simulink model "corde"  (R2019b)
settings: Solver=VariableStepAuto  StartTime=0.0  StopTime=10.0  RelTol=1e-3
libraries: simulink x1
settings Model: Creator=thomaslabbe  LastModifiedBy=thomaslabbe

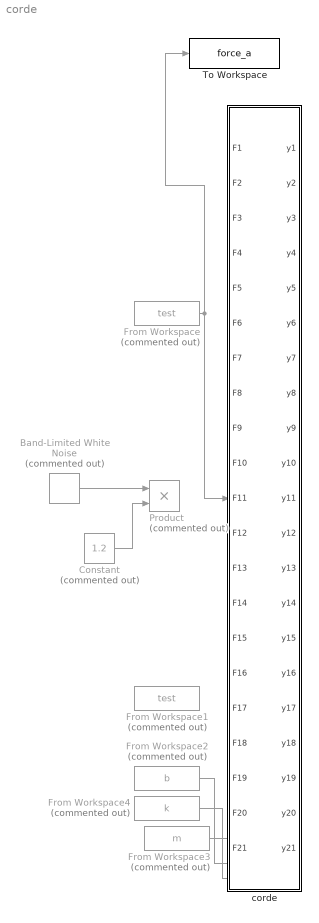
== system corde ==
  Band-Limited White Noise : simulink/Sources/Band-Limited White Noise  Commented=on  Cov=[0.1]  Ts=0.1  seed=[23341]
  Constant : Constant  Commented=on  Value=1.2
  From Workspace : FromWorkspace  Commented=on  VariableName=test  SampleTime=0
  From Workspace1 : FromWorkspace  Commented=on  VariableName=test  SampleTime=0
  From Workspace2 : FromWorkspace  Commented=on  VariableName=b  SampleTime=0
  From Workspace3 : FromWorkspace  Commented=on  VariableName=m  SampleTime=0
  From Workspace4 : FromWorkspace  Commented=on  VariableName=k  SampleTime=0
  Product : Product  Commented=on
  To Workspace : ToWorkspace  VariableName=force_a  SaveFormat=Timeseries  SampleTime=-1
  "corde " : Subsystem
  wires:
  From Workspace4/1 -> ?
  From Workspace3/1 -> ?
  From Workspace2/1 -> ?
  From Workspace/1 -> "corde "/11(F11), To Workspace/1
  Constant/1 -> Product/2
  Band-Limited White Noise/1 -> Product/1

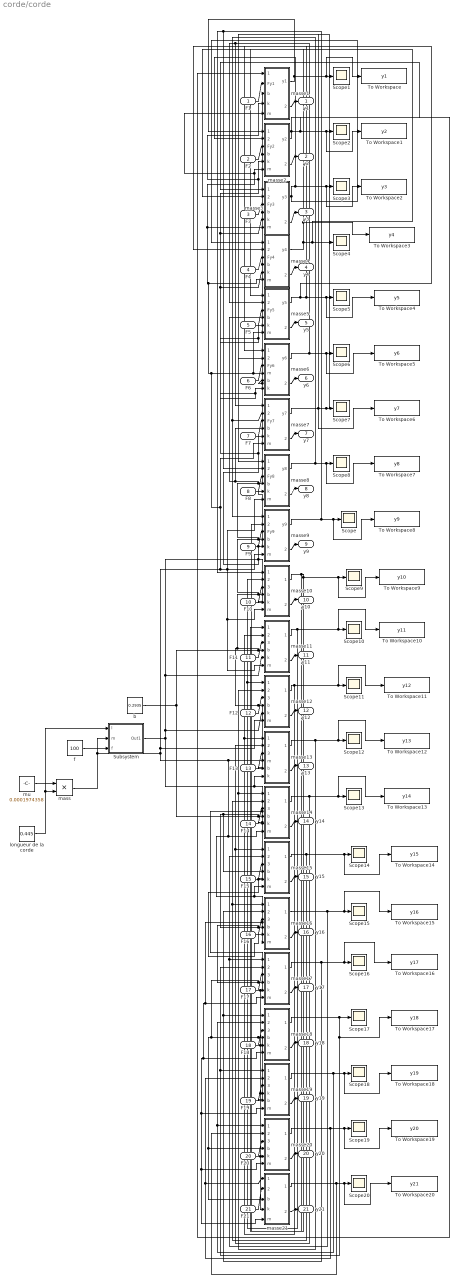
== system corde/corde  ==
  F1 : Inport
  F2 : Inport  Port=2
  F3 : Inport  Port=3
  F4 : Inport  Port=4
  F5 : Inport  Port=5
  F6 : Inport  Port=6
  F7 : Inport  Port=7
  F8 : Inport  Port=8
  F9 : Inport  Port=9
  F10 : Inport  Port=10
  F11 : Inport  Port=11
  F12 : Inport  Port=12
  F13 : Inport  Port=13
  F14 : Inport  Port=14
  F15 : Inport  Port=15
  F16 : Inport  Port=16
  F17 : Inport  Port=17
  F18 : Inport  Port=18
  F19 : Inport  Port=19
  F20 : Inport  Port=20
  F21 : Inport  Port=21
  Scope{,1..20} (21 alike) : Scope
  Subsystem : Subsystem
  To Workspace : ToWorkspace  VariableName=y1  SampleTime=-1
      settings: Save2DSignal=2-D array (concatenate along first dimension)
  To Workspace1 : ToWorkspace  VariableName=y2  SampleTime=-1
      settings: Save2DSignal=2-D array (concatenate along first dimension)
  To Workspace10 : ToWorkspace  VariableName=y11  SampleTime=-1
      settings: Save2DSignal=2-D array (concatenate along first dimension)
  To Workspace11 : ToWorkspace  VariableName=y12  SampleTime=-1
      settings: Save2DSignal=2-D array (concatenate along first dimension)
  To Workspace12 : ToWorkspace  VariableName=y13  SampleTime=-1
      settings: Save2DSignal=2-D array (concatenate along first dimension)
  To Workspace13 : ToWorkspace  VariableName=y14  SampleTime=-1
      settings: Save2DSignal=2-D array (concatenate along first dimension)
  To Workspace14 : ToWorkspace  VariableName=y15  SampleTime=-1
      settings: Save2DSignal=2-D array (concatenate along first dimension)
  To Workspace15 : ToWorkspace  VariableName=y16  SampleTime=-1
      settings: Save2DSignal=2-D array (concatenate along first dimension)
  To Workspace16 : ToWorkspace  VariableName=y17  SampleTime=-1
      settings: Save2DSignal=2-D array (concatenate along first dimension)
  To Workspace17 : ToWorkspace  VariableName=y18  SampleTime=-1
      settings: Save2DSignal=2-D array (concatenate along first dimension)
  To Workspace18 : ToWorkspace  VariableName=y19  SampleTime=-1
      settings: Save2DSignal=2-D array (concatenate along first dimension)
  To Workspace19 : ToWorkspace  VariableName=y20  SampleTime=-1
      settings: Save2DSignal=2-D array (concatenate along first dimension)
  To Workspace2 : ToWorkspace  VariableName=y3  SampleTime=-1
      settings: Save2DSignal=2-D array (concatenate along first dimension)
  To Workspace20 : ToWorkspace  VariableName=y21  SampleTime=-1
      settings: Save2DSignal=2-D array (concatenate along first dimension)
  To Workspace3 : ToWorkspace  VariableName=y4  SampleTime=-1
      settings: Save2DSignal=2-D array (concatenate along first dimension)
  To Workspace4 : ToWorkspace  VariableName=y5  SampleTime=-1
      settings: Save2DSignal=2-D array (concatenate along first dimension)
  To Workspace5 : ToWorkspace  VariableName=y6  SampleTime=-1
      settings: Save2DSignal=2-D array (concatenate along first dimension)
  To Workspace6 : ToWorkspace  VariableName=y7  SampleTime=-1
      settings: Save2DSignal=2-D array (concatenate along first dimension)
  To Workspace7 : ToWorkspace  VariableName=y8  SampleTime=-1
      settings: Save2DSignal=2-D array (concatenate along first dimension)
  To Workspace8 : ToWorkspace  VariableName=y9  SampleTime=-1
      settings: Save2DSignal=2-D array (concatenate along first dimension)
  To Workspace9 : ToWorkspace  VariableName=y10  SampleTime=-1
      settings: Save2DSignal=2-D array (concatenate along first dimension)
  b : Constant  Value=0.2935
  f : Constant  Value=100
  "longueur de la corde " : Constant  Value=0.445
  mass : Product
  masse1 : Subsystem  mask{m=0.01, k=2000, b=0.1, pos_ini=0, v_ini=0}
      mask prompts: m "Masse"; k "Force rappel d'un ressort"; b "Frottement"; pos_ini "Position initiale"; v_ini "Vitesse initiale"
  masse10 : Subsystem  mask{m=0.01, k=2000, b=0.1, pos_ini=0, v_ini=0}
      mask prompts: m "Masse"; k "Force rappel d'un ressort"; b "Frottement"; pos_ini "Position initiale"; v_ini "Vitesse initiale"
  masse11 : Subsystem  mask{m=0.01, k=2000, b=0.1, pos_ini=0, v_ini=0}
      mask prompts: m "Masse"; k "Force rappel d'un ressort"; b "Frottement"; pos_ini "Position initiale"; v_ini "Vitesse initiale"
  masse12 : Subsystem  mask{m=0.01, k=2000, b=0.1, pos_ini=0, v_ini=0}
      mask prompts: m "Masse"; k "Force rappel d'un ressort"; b "Frottement"; pos_ini "Position initiale"; v_ini "Vitesse initiale"
  masse13 : Subsystem  mask{m=0.01, k=2000, b=0.1, pos_ini=0, v_ini=0}
      mask prompts: m "Masse"; k "Force rappel d'un ressort"; b "Frottement"; pos_ini "Position initiale"; v_ini "Vitesse initiale"
  masse14 : Subsystem  mask{m=0.01, k=2000, b=0.1, pos_ini=0, v_ini=0}
      mask prompts: m "Masse"; k "Force rappel d'un ressort"; b "Frottement"; pos_ini "Position initiale"; v_ini "Vitesse initiale"
  masse15 : Subsystem  mask{m=0.01, k=2000, b=0.1, pos_ini=0, v_ini=0}
      mask prompts: m "Masse"; k "Force rappel d'un ressort"; b "Frottement"; pos_ini "Position initiale"; v_ini "Vitesse initiale"
  masse16 : Subsystem  mask{m=0.01, k=2000, b=0.1, pos_ini=0, v_ini=0}
      mask prompts: m "Masse"; k "Force rappel d'un ressort"; b "Frottement"; pos_ini "Position initiale"; v_ini "Vitesse initiale"
  masse17 : Subsystem  mask{m=0.01, k=2000, b=0.1, pos_ini=0, v_ini=0}
      mask prompts: m "Masse"; k "Force rappel d'un ressort"; b "Frottement"; pos_ini "Position initiale"; v_ini "Vitesse initiale"
  masse18 : Subsystem  mask{m=0.01, k=2000, b=0.1, pos_ini=0, v_ini=0}
      mask prompts: m "Masse"; k "Force rappel d'un ressort"; b "Frottement"; pos_ini "Position initiale"; v_ini "Vitesse initiale"
  masse19 : Subsystem  mask{m=0.01, k=2000, b=0.1, pos_ini=0, v_ini=0}
      mask prompts: m "Masse"; k "Force rappel d'un ressort"; b "Frottement"; pos_ini "Position initiale"; v_ini "Vitesse initiale"
  "masse2 " : Subsystem  mask{m=0.01, k=2000, b=0.1, pos_ini=0, v_ini=0}
      mask prompts: m "Masse"; k "Force rappel d'un ressort"; b "Frottement"; pos_ini "Position initiale"; v_ini "Vitesse initiale"
  masse20 : Subsystem  mask{m=0.01, k=2000, b=0.1, pos_ini=0, v_ini=0}
      mask prompts: m "Masse"; k "Force rappel d'un ressort"; b "Frottement"; pos_ini "Position initiale"; v_ini "Vitesse initiale"
  masse21 : Subsystem  mask{m=0.01, k=2000, b=0.1, pos_ini=0.0, v_ini=0}
      mask prompts: m "Masse"; k "Force rappel d'un ressort"; b "Frottement"; pos_ini "Position initiale"; v_ini "Vitesse initiale"
  masse3 : Subsystem  mask{m=0.01, k=2000, b=0.1, pos_ini=0, v_ini=0}
      mask prompts: m "Masse"; k "Force rappel d'un ressort"; b "Frottement"; pos_ini "Position initiale"; v_ini "Vitesse initiale"
  masse4 : Subsystem  mask{m=0.01, k=2000, b=0.1, pos_ini=0, v_ini=0}
      mask prompts: m "Masse"; k "Force rappel d'un ressort"; b "Frottement"; pos_ini "Position initiale"; v_ini "Vitesse initiale"
  masse5 : Subsystem  mask{m=0.01, k=2000, b=0.1, pos_ini=0, v_ini=0}
      mask prompts: m "Masse"; k "Force rappel d'un ressort"; b "Frottement"; pos_ini "Position initiale"; v_ini "Vitesse initiale"
  masse6 : Subsystem  mask{m=0.01, k=2000, b=0.1, pos_ini=0, v_ini=0}
      mask prompts: m "Masse"; k "Force rappel d'un ressort"; b "Frottement"; pos_ini "Position initiale"; v_ini "Vitesse initiale"
  masse7 : Subsystem  mask{m=0.01, k=2000, b=0.1, pos_ini=0, v_ini=0}
      mask prompts: m "Masse"; k "Force rappel d'un ressort"; b "Frottement"; pos_ini "Position initiale"; v_ini "Vitesse initiale"
  masse8 : Subsystem  mask{m=0.01, k=2000, b=0.1, pos_ini=0, v_ini=0}
      mask prompts: m "Masse"; k "Force rappel d'un ressort"; b "Frottement"; pos_ini "Position initiale"; v_ini "Vitesse initiale"
  masse9 : Subsystem  mask{m=0.01, k=2000, b=0.1, pos_ini=0, v_ini=0}
      mask prompts: m "Masse"; k "Force rappel d'un ressort"; b "Frottement"; pos_ini "Position initiale"; v_ini "Vitesse initiale"
  mu : Constant  Value=0.0001974358
  y1 : Outport
  y2 : Outport  Port=2
  y3 : Outport  Port=3
  y4 : Outport  Port=4
  y5 : Outport  Port=5
  y6 : Outport  Port=6
  y7 : Outport  Port=7
  y8 : Outport  Port=8
  y9 : Outport  Port=9
  y10 : Outport  Port=10
  y11 : Outport  Port=11
  y12 : Outport  Port=12
  y13 : Outport  Port=13
  y14 : Outport  Port=14
  y15 : Outport  Port=15
  y16 : Outport  Port=16
  y17 : Outport  Port=17
  y18 : Outport  Port=18
  y19 : Outport  Port=19
  y20 : Outport  Port=20
  y21 : Outport  Port=21
  wires:
  masse20/2(vy20) -> y20/1
  masse8/2(vy8) -> y8/1
  masse4/2(vy4) -> y4/1
  masse17/2(vy17) -> y17/1
  F17/1 -> masse17/3(Fy17)
  F1/1 -> masse1/2(Fy1)
  F5/1 -> masse5/3(Fy5)
  masse7/2(vy7) -> y7/1
  masse19/2(vy19) -> y19/1
  "masse2 "/2(vy2) -> y2/1
  F21/1 -> masse21/2(Fy21)
  F10/1 -> masse10/3(Fy10)
  masse15/1(y15) -> To Workspace14/1, Scope14/1, masse16/1(yp15), masse14/2(yp15)
  F11/1 -> masse11/3(Fy11)
  F6/1 -> masse6/3(Fy6)
  F15/1 -> masse15/3(Fy15)
  masse1/2(vy1) -> y1/1
  masse10/2(vy10) -> y10/1
  "masse2 "/1(y2) -> masse3/1(yp2), To Workspace1/1, Scope2/1, masse1/1(yp2)
  F2/1 -> "masse2 "/3(Fy2)
  F14/1 -> masse14/3(Fy14)
  masse17/1(y17) -> To Workspace16/1, Scope16/1, masse18/1(yp17), masse16/2(yp17)
  masse12/2(vy12) -> y12/1
  F4/1 -> masse4/3(Fy4)
  masse6/2(vy6) -> y6/1
  masse19/1(y19) -> To Workspace18/1, Scope18/1, masse20/1(yp19), masse18/2(yp19)
  masse5/1(y5) -> masse4/2(yp5), To Workspace4/1, Scope5/1, masse6/1(yp5)
  masse3/2(vy3) -> y3/1
  masse16/2(vy16) -> y16/1
  masse11/2(vy11) -> y11/1
  masse13/1(y13) -> To Workspace12/1, Scope12/1, masse14/1(yp13), masse12/2(yp13)
  masse12/1(y12) -> To Workspace11/1, Scope11/1, masse13/1(yp12), masse11/2(yp12)
  F20/1 -> masse20/3(Fy20)
  F18/1 -> masse18/3(Fy18)
  masse18/2(vy18) -> y18/1
  masse8/1(y8) -> To Workspace7/1, Scope8/1, masse9/1(yp8), masse7/2(yp8)
  masse21/2(vy21) -> y21/1
  masse9/2(vy9) -> y9/1
  masse14/1(y14) -> To Workspace13/1, Scope13/1, masse15/1(yp14), masse13/2(yp14)
  masse20/1(y20) -> To Workspace19/1, Scope19/1, masse21/1(yp20), masse19/2(yp20)
  F19/1 -> masse19/3(Fy19)
  masse16/1(y16) -> To Workspace15/1, Scope15/1, masse17/1(yp16), masse15/2(yp16)
  masse9/1(y9) -> masse8/2(yp9), masse10/1(yp9), To Workspace8/1, Scope/1
  masse5/2(vy5) -> y5/1
  masse11/1(y11) -> To Workspace10/1, Scope10/1, masse12/1(yp11), masse10/2(yp11)
  masse3/1(y3) -> To Workspace2/1, Scope3/1, "masse2 "/2(yp3), masse4/1(yp3)
  masse21/1(y21) -> To Workspace20/1, Scope20/1, masse20/2(yp21)
  F8/1 -> masse8/3(Fy8)
  masse13/2(vy13) -> y13/1
  F9/1 -> masse9/3(Fy9)
  masse10/1(y10) -> masse9/2(yp10), To Workspace9/1, Scope9/1, masse11/1(yp10)
  F16/1 -> masse16/3(Fy16)
  masse18/1(y18) -> masse19/1(yp18), masse17/2(yp18), To Workspace17/1, Scope17/1
  masse6/1(y6) -> masse7/1(yp6), masse5/2(yp6), To Workspace5/1, Scope6/1
  F7/1 -> masse7/3(Fy7)
  F13/1 -> masse13/3(Fy13)
  masse4/1(y4) -> masse5/1(yp4), To Workspace3/1, masse3/2(yp4), Scope4/1
  F12/1 -> masse12/3(Fy12)
  masse15/2(vy15) -> y15/1
  F3/1 -> masse3/3(Fy3)
  masse7/1(y7) -> masse6/2(yp7), Scope7/1, masse8/1(yp7), To Workspace6/1
  masse14/2(vy14) -> y14/1
  masse1/1(y1) -> To Workspace/1, Scope1/1, "masse2 "/1(yp1)
  b/1 -> masse15/4(b), masse19/5(b), masse18/4(b), masse20/4(b), masse21/3(b), masse17/4(b), masse16/4(b), masse14/4(b), masse6/5("b "), masse1/3(b), "masse2 "/4(b), masse3/4(b), masse4/4(b), masse7/4(b), masse5/4("b "), masse8/4(b), masse9/4(b), masse10/4(b), masse13/5(b), masse12/4(b), masse11/4(b)
  mass/1 -> Subsystem/2(m), masse7/6(m), masse6/4(m), masse5/6(m), masse4/6(m), masse3/6(m), "masse2 "/6(m), masse1/5(m), masse10/6(m), masse11/6(m), masse9/6(m), masse8/6(m), masse12/6(m), masse13/4(m), masse14/6(m), masse16/6(m), masse17/6(m), masse18/6(m), masse19/6(m), masse20/6(m), masse21/5(m), masse15/6(m)
  Subsystem/1(Out1) -> masse8/5(k), masse9/5(k), masse7/5(k), masse6/6(k), masse5/5(k), masse4/5(k), masse3/5(k), "masse2 "/5(k), masse1/4(k), masse10/5(k), masse11/5(k), masse12/5(k), masse14/5("k "), masse16/5(k), masse15/5(k), masse21/4(k), masse20/5(k), masse19/4(k), masse18/5(k), masse17/5(k), masse13/6(k)
  f/1 -> Subsystem/3(f)
  "longueur de la corde "/1 -> Subsystem/1(l), mass/2
  mu/1 -> mass/1

== system corde/corde /Subsystem ==
  l : Inport
  m : Inport  Port=2
  f : Inport  Port=3
  Divide : Product  Inputs=*/
  Divide1 : Product  Inputs=*/
  Sqrt : Sqrt  SaturateOnIntegerOverflow=on
  Tension : Polyval  Coefs=[1.138, -56.541]
  Out1 : Outport
  wires:
  Sqrt/1 -> Out1/1
  f/1 -> Tension/1
  Divide1/1 -> Sqrt/1
  Tension/1 -> Divide/1
  l/1 -> Divide/2
  Divide/1 -> Divide1/1
  m/1 -> Divide1/2

== system corde/corde /masse1 ==
  yp2 : Inport
  Fy1 : Inport  Port=2
  b : Inport  Port=3
  k : Inport  Port=4
  m : Inport  Port=5
  " " : Gain  Gain=2  SaturateOnIntegerOverflow=on  OutDataTypeStr=Inherit: Same as input  ParamDataTypeStr=Inherit: Same as input
  Divide : Product  Inputs=*/
  Position y1 : Integrator  InitialCondition=pos_ini
  Product1 : Product
  Product2 : Product
  Somme Force : Sum  Inputs=++-  SaturateOnIntegerOverflow=on  InputSameDT=on  OutDataTypeStr=Inherit: Same as first input
  Somme y : Sum  Inputs=-+  SaturateOnIntegerOverflow=on  InputSameDT=on  OutDataTypeStr=Inherit: Same as first input
  Vitesse y1 : Integrator  InitialCondition=v_ini
  y1 : Outport  VectorParamsAs1DForOutWhenUnconnected=off
  vy1 : Outport  Port=2  VectorParamsAs1DForOutWhenUnconnected=off
  wires:
  Position y1/1 -> " "/1, y1/1
  Vitesse y1/1 -> Position y1/1, Product2/2, vy1/1
  Divide/1 -> Vitesse y1/1
  Somme Force/1 -> Divide/1
  Product1/1 -> Somme Force/1
  Somme y/1 -> Product1/2
  Product2/1 -> Somme Force/3
  Fy1/1 -> Somme Force/2
  yp2/1 -> Somme y/2
  " "/1 -> Somme y/1
  b/1 -> Product2/1
  k/1 -> Product1/1
  m/1 -> Divide/2

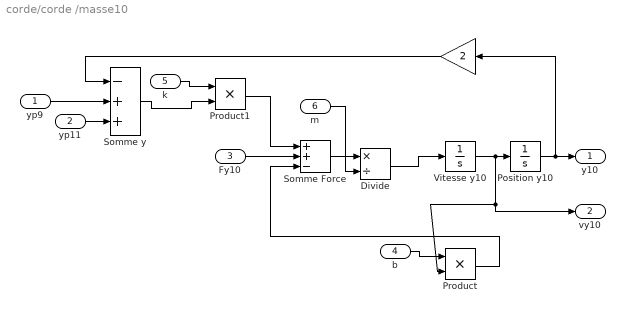
== system corde/corde /masse10 ==
  yp9 : Inport
  yp11 : Inport  Port=2
  Fy10 : Inport  Port=3
  b : Inport  Port=4
  k : Inport  Port=5
  m : Inport  Port=6
  " " : Gain  Gain=2  SaturateOnIntegerOverflow=on  OutDataTypeStr=Inherit: Same as input  ParamDataTypeStr=Inherit: Same as input
  Divide : Product  Inputs=*/
  Position y10 : Integrator  InitialCondition=pos_ini
  Product : Product
  Product1 : Product
  Somme Force : Sum  Inputs=++-  SaturateOnIntegerOverflow=on  InputSameDT=on  OutDataTypeStr=Inherit: Same as first input
  Somme y : Sum  Inputs=-++  SaturateOnIntegerOverflow=on  InputSameDT=on  OutDataTypeStr=Inherit: Same as first input
  Vitesse y10 : Integrator  InitialCondition=v_ini
  y10 : Outport  VectorParamsAs1DForOutWhenUnconnected=off
  vy10 : Outport  Port=2  VectorParamsAs1DForOutWhenUnconnected=off
  wires:
  Position y10/1 -> " "/1, y10/1
  Vitesse y10/1 -> Position y10/1, vy10/1, Product/2
  Divide/1 -> Vitesse y10/1
  Somme Force/1 -> Divide/1
  Product1/1 -> Somme Force/1
  Somme y/1 -> Product1/2
  Product/1 -> Somme Force/3
  Fy10/1 -> Somme Force/2
  yp11/1 -> Somme y/3
  yp9/1 -> Somme y/2
  " "/1 -> Somme y/1
  b/1 -> Product/1
  k/1 -> Product1/1
  m/1 -> Divide/2

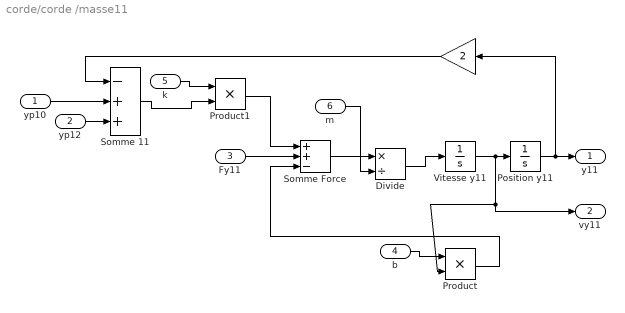
== system corde/corde /masse11 ==
  yp10 : Inport
  yp12 : Inport  Port=2
  Fy11 : Inport  Port=3
  b : Inport  Port=4
  k : Inport  Port=5
  m : Inport  Port=6
  " " : Gain  Gain=2  SaturateOnIntegerOverflow=on  OutDataTypeStr=Inherit: Same as input  ParamDataTypeStr=Inherit: Same as input
  Divide : Product  Inputs=*/
  Position y11 : Integrator  InitialCondition=pos_ini
  Product : Product
  Product1 : Product
  Somme 11 : Sum  Inputs=-++  SaturateOnIntegerOverflow=on  InputSameDT=on  OutDataTypeStr=Inherit: Same as first input
  Somme Force : Sum  Inputs=++-  SaturateOnIntegerOverflow=on  InputSameDT=on  OutDataTypeStr=Inherit: Same as first input
  Vitesse y11 : Integrator  InitialCondition=v_ini
  y11 : Outport  VectorParamsAs1DForOutWhenUnconnected=off
  vy11 : Outport  Port=2  VectorParamsAs1DForOutWhenUnconnected=off
  wires:
  Position y11/1 -> " "/1, y11/1
  Vitesse y11/1 -> Position y11/1, vy11/1, Product/2
  Divide/1 -> Vitesse y11/1
  Somme Force/1 -> Divide/1
  Product1/1 -> Somme Force/1
  Somme 11/1 -> Product1/2
  Product/1 -> Somme Force/3
  Fy11/1 -> Somme Force/2
  yp12/1 -> Somme 11/3
  yp10/1 -> Somme 11/2
  " "/1 -> Somme 11/1
  b/1 -> Product/1
  k/1 -> Product1/1
  m/1 -> Divide/2

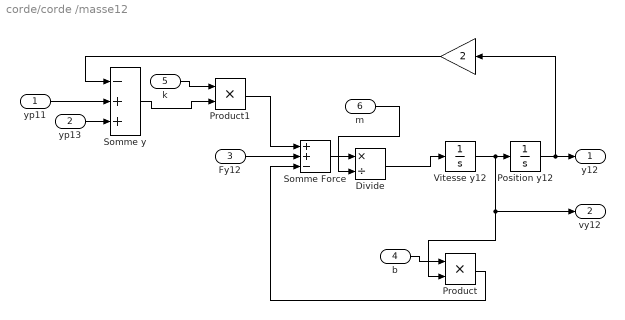
== system corde/corde /masse12 ==
  yp11 : Inport
  yp13 : Inport  Port=2
  Fy12 : Inport  Port=3
  b : Inport  Port=4
  k : Inport  Port=5
  m : Inport  Port=6
  " " : Gain  Gain=2  SaturateOnIntegerOverflow=on  OutDataTypeStr=Inherit: Same as input  ParamDataTypeStr=Inherit: Same as input
  Divide : Product  Inputs=*/
  Position y12 : Integrator  InitialCondition=pos_ini
  Product : Product
  Product1 : Product
  Somme Force : Sum  Inputs=++-  SaturateOnIntegerOverflow=on  InputSameDT=on  OutDataTypeStr=Inherit: Same as first input
  Somme y : Sum  Inputs=-++  SaturateOnIntegerOverflow=on  InputSameDT=on  OutDataTypeStr=Inherit: Same as first input
  Vitesse y12 : Integrator  InitialCondition=v_ini
  y12 : Outport  VectorParamsAs1DForOutWhenUnconnected=off
  vy12 : Outport  Port=2  VectorParamsAs1DForOutWhenUnconnected=off
  wires:
  Position y12/1 -> " "/1, y12/1
  Vitesse y12/1 -> Position y12/1, Product/2, vy12/1
  Divide/1 -> Vitesse y12/1
  Somme Force/1 -> Divide/1
  Product1/1 -> Somme Force/1
  Somme y/1 -> Product1/2
  Product/1 -> Somme Force/3
  Fy12/1 -> Somme Force/2
  yp13/1 -> Somme y/3
  yp11/1 -> Somme y/2
  " "/1 -> Somme y/1
  b/1 -> Product/1
  k/1 -> Product1/1
  m/1 -> Divide/2

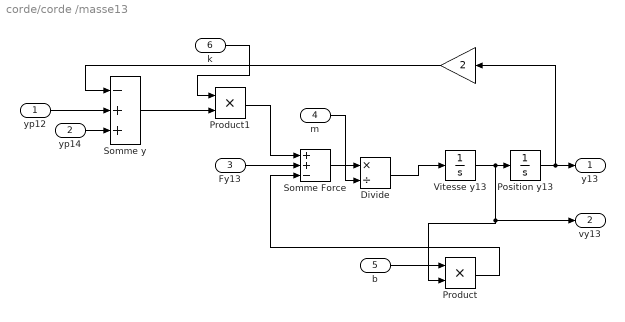
== system corde/corde /masse13 ==
  yp12 : Inport
  yp14 : Inport  Port=2
  Fy13 : Inport  Port=3
  m : Inport  Port=4
  b : Inport  Port=5
  k : Inport  Port=6
  " " : Gain  Gain=2  SaturateOnIntegerOverflow=on  OutDataTypeStr=Inherit: Same as input  ParamDataTypeStr=Inherit: Same as input
  Divide : Product  Inputs=*/
  Position y13 : Integrator  InitialCondition=pos_ini
  Product : Product
  Product1 : Product
  Somme Force : Sum  Inputs=++-  SaturateOnIntegerOverflow=on  InputSameDT=on  OutDataTypeStr=Inherit: Same as first input
  Somme y : Sum  Inputs=-++  SaturateOnIntegerOverflow=on  InputSameDT=on  OutDataTypeStr=Inherit: Same as first input
  Vitesse y13 : Integrator  InitialCondition=v_ini
  y13 : Outport  VectorParamsAs1DForOutWhenUnconnected=off
  vy13 : Outport  Port=2  VectorParamsAs1DForOutWhenUnconnected=off
  wires:
  Position y13/1 -> " "/1, y13/1
  Vitesse y13/1 -> Position y13/1, Product/2, vy13/1
  Divide/1 -> Vitesse y13/1
  Somme Force/1 -> Divide/1
  Product1/1 -> Somme Force/1
  Somme y/1 -> Product1/2
  Product/1 -> Somme Force/3
  Fy13/1 -> Somme Force/2
  yp14/1 -> Somme y/3
  yp12/1 -> Somme y/2
  " "/1 -> Somme y/1
  m/1 -> Divide/2
  b/1 -> Product/1
  k/1 -> Product1/1

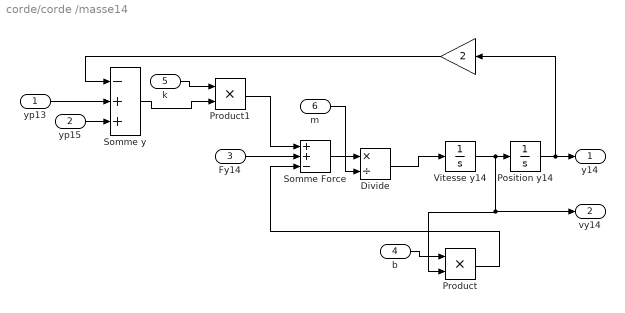
== system corde/corde /masse14 ==
  yp13 : Inport
  yp15 : Inport  Port=2
  Fy14 : Inport  Port=3
  b : Inport  Port=4
  "k " : Inport  Port=5
  m : Inport  Port=6
  " " : Gain  Gain=2  SaturateOnIntegerOverflow=on  OutDataTypeStr=Inherit: Same as input  ParamDataTypeStr=Inherit: Same as input
  Divide : Product  Inputs=*/
  Position y14 : Integrator  InitialCondition=pos_ini
  Product : Product
  Product1 : Product
  Somme Force : Sum  Inputs=++-  SaturateOnIntegerOverflow=on  InputSameDT=on  OutDataTypeStr=Inherit: Same as first input
  Somme y : Sum  Inputs=-++  SaturateOnIntegerOverflow=on  InputSameDT=on  OutDataTypeStr=Inherit: Same as first input
  Vitesse y14 : Integrator  InitialCondition=v_ini
  y14 : Outport  VectorParamsAs1DForOutWhenUnconnected=off
  vy14 : Outport  Port=2  VectorParamsAs1DForOutWhenUnconnected=off
  wires:
  Position y14/1 -> " "/1, y14/1
  Vitesse y14/1 -> Position y14/1, Product/2, vy14/1
  Divide/1 -> Vitesse y14/1
  Somme Force/1 -> Divide/1
  Product1/1 -> Somme Force/1
  Somme y/1 -> Product1/2
  Product/1 -> Somme Force/3
  Fy14/1 -> Somme Force/2
  yp15/1 -> Somme y/3
  yp13/1 -> Somme y/2
  " "/1 -> Somme y/1
  b/1 -> Product/1
  "k "/1 -> Product1/1
  m/1 -> Divide/2

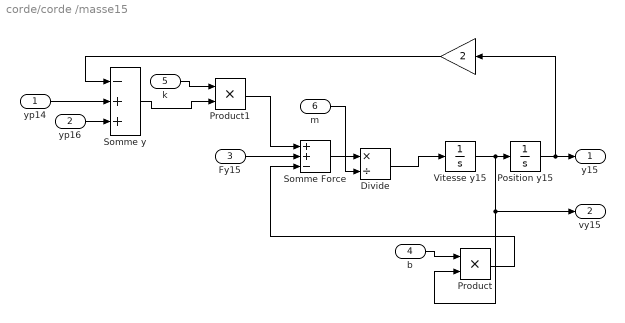
== system corde/corde /masse15 ==
  yp14 : Inport
  yp16 : Inport  Port=2
  Fy15 : Inport  Port=3
  b : Inport  Port=4
  k : Inport  Port=5
  m : Inport  Port=6
  " " : Gain  Gain=2  SaturateOnIntegerOverflow=on  OutDataTypeStr=Inherit: Same as input  ParamDataTypeStr=Inherit: Same as input
  Divide : Product  Inputs=*/
  Position y15 : Integrator  InitialCondition=pos_ini
  Product : Product
  Product1 : Product
  Somme Force : Sum  Inputs=++-  SaturateOnIntegerOverflow=on  InputSameDT=on  OutDataTypeStr=Inherit: Same as first input
  Somme y : Sum  Inputs=-++  SaturateOnIntegerOverflow=on  InputSameDT=on  OutDataTypeStr=Inherit: Same as first input
  Vitesse y15 : Integrator  InitialCondition=v_ini
  y15 : Outport  VectorParamsAs1DForOutWhenUnconnected=off
  vy15 : Outport  Port=2  VectorParamsAs1DForOutWhenUnconnected=off
  wires:
  Position y15/1 -> " "/1, y15/1
  Vitesse y15/1 -> Position y15/1, Product/2, vy15/1
  Divide/1 -> Vitesse y15/1
  Somme Force/1 -> Divide/1
  Product1/1 -> Somme Force/1
  Somme y/1 -> Product1/2
  Product/1 -> Somme Force/3
  Fy15/1 -> Somme Force/2
  yp16/1 -> Somme y/3
  yp14/1 -> Somme y/2
  " "/1 -> Somme y/1
  b/1 -> Product/1
  k/1 -> Product1/1
  m/1 -> Divide/2

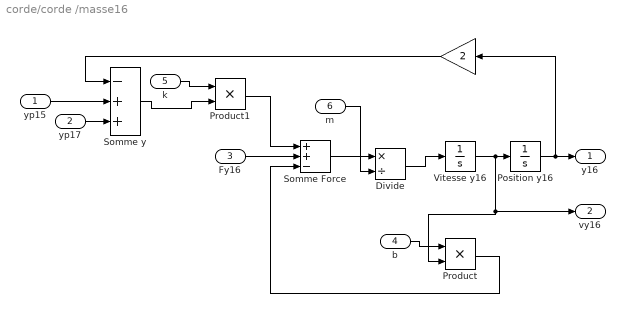
== system corde/corde /masse16 ==
  yp15 : Inport
  yp17 : Inport  Port=2
  Fy16 : Inport  Port=3
  b : Inport  Port=4
  k : Inport  Port=5
  m : Inport  Port=6
  " " : Gain  Gain=2  SaturateOnIntegerOverflow=on  OutDataTypeStr=Inherit: Same as input  ParamDataTypeStr=Inherit: Same as input
  Divide : Product  Inputs=*/
  Position y16 : Integrator  InitialCondition=pos_ini
  Product : Product
  Product1 : Product
  Somme Force : Sum  Inputs=++-  SaturateOnIntegerOverflow=on  InputSameDT=on  OutDataTypeStr=Inherit: Same as first input
  Somme y : Sum  Inputs=-++  SaturateOnIntegerOverflow=on  InputSameDT=on  OutDataTypeStr=Inherit: Same as first input
  Vitesse y16 : Integrator  InitialCondition=v_ini
  y16 : Outport  VectorParamsAs1DForOutWhenUnconnected=off
  vy16 : Outport  Port=2  VectorParamsAs1DForOutWhenUnconnected=off
  wires:
  Position y16/1 -> " "/1, y16/1
  Vitesse y16/1 -> Position y16/1, Product/2, vy16/1
  Divide/1 -> Vitesse y16/1
  Somme Force/1 -> Divide/1
  Product1/1 -> Somme Force/1
  Somme y/1 -> Product1/2
  Product/1 -> Somme Force/3
  Fy16/1 -> Somme Force/2
  yp17/1 -> Somme y/3
  yp15/1 -> Somme y/2
  " "/1 -> Somme y/1
  b/1 -> Product/1
  k/1 -> Product1/1
  m/1 -> Divide/2

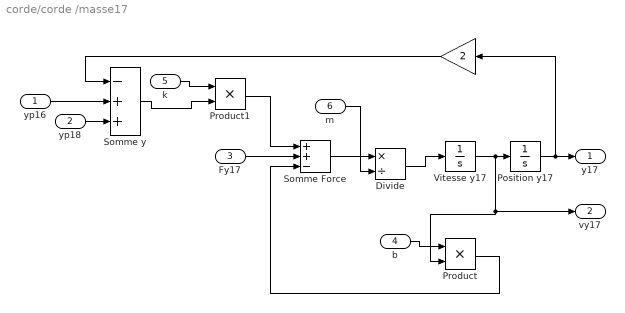
== system corde/corde /masse17 ==
  yp16 : Inport
  yp18 : Inport  Port=2
  Fy17 : Inport  Port=3
  b : Inport  Port=4
  k : Inport  Port=5
  m : Inport  Port=6
  " " : Gain  Gain=2  SaturateOnIntegerOverflow=on  OutDataTypeStr=Inherit: Same as input  ParamDataTypeStr=Inherit: Same as input
  Divide : Product  Inputs=*/
  Position y17 : Integrator  InitialCondition=pos_ini
  Product : Product
  Product1 : Product
  Somme Force : Sum  Inputs=++-  SaturateOnIntegerOverflow=on  InputSameDT=on  OutDataTypeStr=Inherit: Same as first input
  Somme y : Sum  Inputs=-++  SaturateOnIntegerOverflow=on  InputSameDT=on  OutDataTypeStr=Inherit: Same as first input
  Vitesse y17 : Integrator  InitialCondition=v_ini
  y17 : Outport  VectorParamsAs1DForOutWhenUnconnected=off
  vy17 : Outport  Port=2  VectorParamsAs1DForOutWhenUnconnected=off
  wires:
  Position y17/1 -> " "/1, y17/1
  Vitesse y17/1 -> Position y17/1, Product/2, vy17/1
  Divide/1 -> Vitesse y17/1
  Somme Force/1 -> Divide/1
  Product1/1 -> Somme Force/1
  Somme y/1 -> Product1/2
  Product/1 -> Somme Force/3
  Fy17/1 -> Somme Force/2
  yp18/1 -> Somme y/3
  yp16/1 -> Somme y/2
  " "/1 -> Somme y/1
  b/1 -> Product/1
  k/1 -> Product1/1
  m/1 -> Divide/2

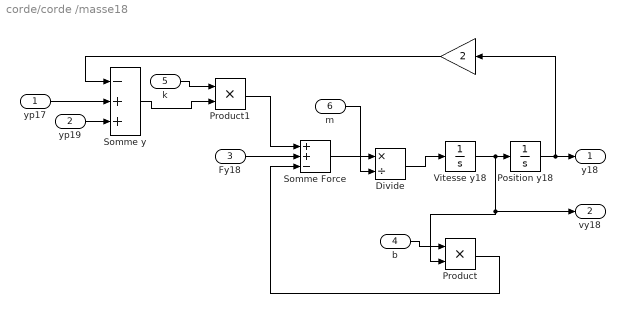
== system corde/corde /masse18 ==
  yp17 : Inport
  yp19 : Inport  Port=2
  Fy18 : Inport  Port=3
  b : Inport  Port=4
  k : Inport  Port=5
  m : Inport  Port=6
  " " : Gain  Gain=2  SaturateOnIntegerOverflow=on  OutDataTypeStr=Inherit: Same as input  ParamDataTypeStr=Inherit: Same as input
  Divide : Product  Inputs=*/
  Position y18 : Integrator  InitialCondition=pos_ini
  Product : Product
  Product1 : Product
  Somme Force : Sum  Inputs=++-  SaturateOnIntegerOverflow=on  InputSameDT=on  OutDataTypeStr=Inherit: Same as first input
  Somme y : Sum  Inputs=-++  SaturateOnIntegerOverflow=on  InputSameDT=on  OutDataTypeStr=Inherit: Same as first input
  Vitesse y18 : Integrator  InitialCondition=v_ini
  y18 : Outport  VectorParamsAs1DForOutWhenUnconnected=off
  vy18 : Outport  Port=2  VectorParamsAs1DForOutWhenUnconnected=off
  wires:
  Position y18/1 -> " "/1, y18/1
  Vitesse y18/1 -> Position y18/1, Product/2, vy18/1
  Divide/1 -> Vitesse y18/1
  Somme Force/1 -> Divide/1
  Product1/1 -> Somme Force/1
  Somme y/1 -> Product1/2
  Product/1 -> Somme Force/3
  Fy18/1 -> Somme Force/2
  yp19/1 -> Somme y/3
  yp17/1 -> Somme y/2
  " "/1 -> Somme y/1
  b/1 -> Product/1
  k/1 -> Product1/1
  m/1 -> Divide/2

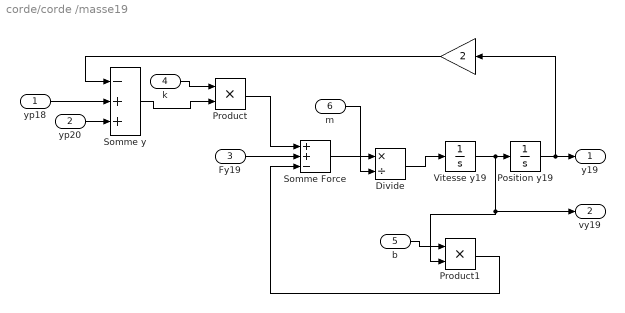
== system corde/corde /masse19 ==
  yp18 : Inport
  yp20 : Inport  Port=2
  Fy19 : Inport  Port=3
  k : Inport  Port=4
  b : Inport  Port=5
  m : Inport  Port=6
  " " : Gain  Gain=2  SaturateOnIntegerOverflow=on  OutDataTypeStr=Inherit: Same as input  ParamDataTypeStr=Inherit: Same as input
  Divide : Product  Inputs=*/
  Position y19 : Integrator  InitialCondition=pos_ini
  Product : Product
  Product1 : Product
  Somme Force : Sum  Inputs=++-  SaturateOnIntegerOverflow=on  InputSameDT=on  OutDataTypeStr=Inherit: Same as first input
  Somme y : Sum  Inputs=-++  SaturateOnIntegerOverflow=on  InputSameDT=on  OutDataTypeStr=Inherit: Same as first input
  Vitesse y19 : Integrator  InitialCondition=v_ini
  y19 : Outport  VectorParamsAs1DForOutWhenUnconnected=off
  vy19 : Outport  Port=2  VectorParamsAs1DForOutWhenUnconnected=off
  wires:
  Position y19/1 -> " "/1, y19/1
  Vitesse y19/1 -> Position y19/1, Product1/2, vy19/1
  Divide/1 -> Vitesse y19/1
  Somme Force/1 -> Divide/1
  Product/1 -> Somme Force/1
  Somme y/1 -> Product/2
  Product1/1 -> Somme Force/3
  Fy19/1 -> Somme Force/2
  yp20/1 -> Somme y/3
  yp18/1 -> Somme y/2
  " "/1 -> Somme y/1
  k/1 -> Product/1
  b/1 -> Product1/1
  m/1 -> Divide/2

== system corde/corde /masse2  ==
  yp1 : Inport
  yp3 : Inport  Port=2
  Fy2 : Inport  Port=3
  b : Inport  Port=4
  k : Inport  Port=5
  m : Inport  Port=6
  " " : Gain  Gain=2  SaturateOnIntegerOverflow=on  OutDataTypeStr=Inherit: Same as input  ParamDataTypeStr=Inherit: Same as input
  Divide : Product  Inputs=*/
  Position y2 : Integrator  InitialCondition=pos_ini
  Product1 : Product
  Product2 : Product
  Somme Force : Sum  Inputs=++-  SaturateOnIntegerOverflow=on  InputSameDT=on  OutDataTypeStr=Inherit: Same as first input
  Somme y : Sum  Inputs=-++  SaturateOnIntegerOverflow=on  InputSameDT=on  OutDataTypeStr=Inherit: Same as first input
  Vitesse y2 : Integrator  InitialCondition=v_ini
  y2 : Outport  VectorParamsAs1DForOutWhenUnconnected=off
  vy2 : Outport  Port=2  VectorParamsAs1DForOutWhenUnconnected=off
  wires:
  Position y2/1 -> " "/1, y2/1
  Vitesse y2/1 -> Position y2/1, Product2/1, vy2/1
  Divide/1 -> Vitesse y2/1
  Somme Force/1 -> Divide/1
  Product1/1 -> Somme Force/1
  Somme y/1 -> Product1/2
  Product2/1 -> Somme Force/3
  Fy2/1 -> Somme Force/2
  yp3/1 -> Somme y/3
  yp1/1 -> Somme y/2
  " "/1 -> Somme y/1
  b/1 -> Product2/2
  k/1 -> Product1/1
  m/1 -> Divide/2

== system corde/corde /masse20 ==
  yp19 : Inport
  yp21 : Inport  Port=2
  Fy20 : Inport  Port=3
  b : Inport  Port=4
  k : Inport  Port=5
  m : Inport  Port=6
  " " : Gain  Gain=2  SaturateOnIntegerOverflow=on  OutDataTypeStr=Inherit: Same as input  ParamDataTypeStr=Inherit: Same as input
  Divide : Product  Inputs=*/
  Position y20 : Integrator  InitialCondition=pos_ini
  Product : Product
  Product1 : Product
  Somme Force : Sum  Inputs=++-  SaturateOnIntegerOverflow=on  InputSameDT=on  OutDataTypeStr=Inherit: Same as first input
  Somme y : Sum  Inputs=-++  SaturateOnIntegerOverflow=on  InputSameDT=on  OutDataTypeStr=Inherit: Same as first input
  Vitesse y20 : Integrator  InitialCondition=v_ini
  y20 : Outport  VectorParamsAs1DForOutWhenUnconnected=off
  vy20 : Outport  Port=2  VectorParamsAs1DForOutWhenUnconnected=off
  wires:
  Position y20/1 -> " "/1, y20/1
  Vitesse y20/1 -> Position y20/1, Product/2, vy20/1
  Divide/1 -> Vitesse y20/1
  Somme Force/1 -> Divide/1
  Product1/1 -> Somme Force/1
  Somme y/1 -> Product1/2
  Product/1 -> Somme Force/3
  Fy20/1 -> Somme Force/2
  yp21/1 -> Somme y/3
  yp19/1 -> Somme y/2
  " "/1 -> Somme y/1
  b/1 -> Product/1
  k/1 -> Product1/1
  m/1 -> Divide/2

== system corde/corde /masse21 ==
  yp20 : Inport
  Fy21 : Inport  Port=2
  b : Inport  Port=3
  k : Inport  Port=4
  m : Inport  Port=5
  " " : Gain  Gain=2  SaturateOnIntegerOverflow=on  OutDataTypeStr=Inherit: Same as input  ParamDataTypeStr=Inherit: Same as input
  Divide : Product  Inputs=*/
  Position y21 : Integrator  InitialCondition=pos_ini
  Product : Product
  Product1 : Product
  Somme Force : Sum  Inputs=++-  SaturateOnIntegerOverflow=on  InputSameDT=on  OutDataTypeStr=Inherit: Same as first input
  Somme y : Sum  Inputs=-+  SaturateOnIntegerOverflow=on  InputSameDT=on  OutDataTypeStr=Inherit: Same as first input
  Vitesse y21 : Integrator  InitialCondition=v_ini
  y21 : Outport  VectorParamsAs1DForOutWhenUnconnected=off
  vy21 : Outport  Port=2  VectorParamsAs1DForOutWhenUnconnected=off
  wires:
  Position y21/1 -> " "/1, y21/1
  Vitesse y21/1 -> Position y21/1, vy21/1, Product/2
  Divide/1 -> Vitesse y21/1
  Somme Force/1 -> Divide/1
  Product1/1 -> Somme Force/1
  Somme y/1 -> Product1/2
  Product/1 -> Somme Force/3
  Fy21/1 -> Somme Force/2
  yp20/1 -> Somme y/2
  " "/1 -> Somme y/1
  b/1 -> Product/1
  k/1 -> Product1/1
  m/1 -> Divide/2

== system corde/corde /masse3 ==
  yp2 : Inport
  yp4 : Inport  Port=2
  Fy3 : Inport  Port=3
  b : Inport  Port=4
  k : Inport  Port=5
  m : Inport  Port=6
  " " : Gain  Gain=2  SaturateOnIntegerOverflow=on  OutDataTypeStr=Inherit: Same as input  ParamDataTypeStr=Inherit: Same as input
  Divide : Product  Inputs=*/
  Position y3 : Integrator  InitialCondition=pos_ini
  Product1 : Product
  Product2 : Product
  Somme Force : Sum  Inputs=++-  SaturateOnIntegerOverflow=on  InputSameDT=on  OutDataTypeStr=Inherit: Same as first input
  Somme y3 : Sum  Inputs=-++  SaturateOnIntegerOverflow=on  InputSameDT=on  OutDataTypeStr=Inherit: Same as first input
  Vitesse y3 : Integrator  InitialCondition=v_ini
  y3 : Outport  VectorParamsAs1DForOutWhenUnconnected=off
  vy3 : Outport  Port=2  VectorParamsAs1DForOutWhenUnconnected=off
  wires:
  Position y3/1 -> " "/1, y3/1
  Vitesse y3/1 -> Position y3/1, Product2/2, vy3/1
  Divide/1 -> Vitesse y3/1
  Product1/1 -> Somme Force/1
  Somme y3/1 -> Product1/2
  Product2/1 -> Somme Force/3
  Fy3/1 -> Somme Force/2
  yp4/1 -> Somme y3/3
  yp2/1 -> Somme y3/2
  " "/1 -> Somme y3/1
  b/1 -> Product2/1
  k/1 -> Product1/1
  Somme Force/1 -> Divide/1
  m/1 -> Divide/2

== system corde/corde /masse4 ==
  yp3 : Inport
  yp5 : Inport  Port=2
  Fy4 : Inport  Port=3
  b : Inport  Port=4
  k : Inport  Port=5
  m : Inport  Port=6
  " " : Gain  Gain=2  SaturateOnIntegerOverflow=on  OutDataTypeStr=Inherit: Same as input  ParamDataTypeStr=Inherit: Same as input
  Divide : Product  Inputs=*/
  Position y4 : Integrator  InitialCondition=pos_ini
  Product1 : Product
  Product2 : Product
  Somme Force : Sum  Inputs=++-  SaturateOnIntegerOverflow=on  InputSameDT=on  OutDataTypeStr=Inherit: Same as first input
  Somme y : Sum  Inputs=-++  SaturateOnIntegerOverflow=on  InputSameDT=on  OutDataTypeStr=Inherit: Same as first input
  Vitesse y4 : Integrator  InitialCondition=v_ini
  y4 : Outport  VectorParamsAs1DForOutWhenUnconnected=off
  vy4 : Outport  Port=2  VectorParamsAs1DForOutWhenUnconnected=off
  wires:
  Position y4/1 -> " "/1, y4/1
  Vitesse y4/1 -> Position y4/1, Product1/2, vy4/1
  Divide/1 -> Vitesse y4/1
  Somme Force/1 -> Divide/1
  Product2/1 -> Somme Force/1
  Somme y/1 -> Product2/1
  Product1/1 -> Somme Force/3
  Fy4/1 -> Somme Force/2
  yp5/1 -> Somme y/3
  yp3/1 -> Somme y/2
  " "/1 -> Somme y/1
  b/1 -> Product1/1
  k/1 -> Product2/2
  m/1 -> Divide/2

== system corde/corde /masse5 ==
  yp4 : Inport
  yp6 : Inport  Port=2
  Fy5 : Inport  Port=3
  "b " : Inport  Port=4
  k : Inport  Port=5
  m : Inport  Port=6
  " " : Gain  Gain=2  SaturateOnIntegerOverflow=on  OutDataTypeStr=Inherit: Same as input  ParamDataTypeStr=Inherit: Same as input
  Divide : Product  Inputs=*/
  Position y5 : Integrator  InitialCondition=pos_ini
  Product1 : Product
  Product2 : Product
  Somme Force : Sum  Inputs=++-  SaturateOnIntegerOverflow=on  InputSameDT=on  OutDataTypeStr=Inherit: Same as first input
  Somme y : Sum  Inputs=-++  SaturateOnIntegerOverflow=on  InputSameDT=on  OutDataTypeStr=Inherit: Same as first input
  Vitesse y5 : Integrator  InitialCondition=v_ini
  y5 : Outport  VectorParamsAs1DForOutWhenUnconnected=off
  vy5 : Outport  Port=2  VectorParamsAs1DForOutWhenUnconnected=off
  wires:
  Position y5/1 -> " "/1, y5/1
  Vitesse y5/1 -> Position y5/1, Product1/2, vy5/1
  Divide/1 -> Vitesse y5/1
  Somme Force/1 -> Divide/1
  Product2/1 -> Somme Force/1
  Somme y/1 -> Product2/2
  Product1/1 -> Somme Force/3
  Fy5/1 -> Somme Force/2
  yp6/1 -> Somme y/3
  yp4/1 -> Somme y/2
  " "/1 -> Somme y/1
  "b "/1 -> Product1/1
  k/1 -> Product2/1
  m/1 -> Divide/2

== system corde/corde /masse6 ==
  yp5 : Inport
  yp7 : Inport  Port=2
  Fy6 : Inport  Port=3
  m : Inport  Port=4
  "b " : Inport  Port=5
  k : Inport  Port=6
  " " : Gain  Gain=2  SaturateOnIntegerOverflow=on  OutDataTypeStr=Inherit: Same as input  ParamDataTypeStr=Inherit: Same as input
  Divide : Product  Inputs=*/
  Position y6 : Integrator  InitialCondition=pos_ini
  Product1 : Product
  Product2 : Product
  Somme Force : Sum  Inputs=++-  SaturateOnIntegerOverflow=on  InputSameDT=on  OutDataTypeStr=Inherit: Same as first input
  Somme y : Sum  Inputs=-++  SaturateOnIntegerOverflow=on  InputSameDT=on  OutDataTypeStr=Inherit: Same as first input
  Vitesse y6 : Integrator  InitialCondition=v_ini
  y6 : Outport  VectorParamsAs1DForOutWhenUnconnected=off
  vy6 : Outport  Port=2  VectorParamsAs1DForOutWhenUnconnected=off
  wires:
  Position y6/1 -> " "/1, y6/1
  Vitesse y6/1 -> Position y6/1, Product1/2, vy6/1
  Divide/1 -> Vitesse y6/1
  Somme Force/1 -> Divide/1
  Product2/1 -> Somme Force/1
  Somme y/1 -> Product2/2
  Product1/1 -> Somme Force/3
  Fy6/1 -> Somme Force/2
  yp7/1 -> Somme y/3
  yp5/1 -> Somme y/2
  " "/1 -> Somme y/1
  m/1 -> Divide/2
  "b "/1 -> Product1/1
  k/1 -> Product2/1

== system corde/corde /masse7 ==
  yp6 : Inport
  yp8 : Inport  Port=2
  Fy7 : Inport  Port=3
  b : Inport  Port=4
  k : Inport  Port=5
  m : Inport  Port=6
  " " : Gain  Gain=2  SaturateOnIntegerOverflow=on  OutDataTypeStr=Inherit: Same as input  ParamDataTypeStr=Inherit: Same as input
  Divide : Product  Inputs=*/
  Position y7 : Integrator  InitialCondition=pos_ini
  Product1 : Product
  Product2 : Product
  Somme Force : Sum  Inputs=++-  SaturateOnIntegerOverflow=on  InputSameDT=on  OutDataTypeStr=Inherit: Same as first input
  Somme y : Sum  Inputs=-++  SaturateOnIntegerOverflow=on  InputSameDT=on  OutDataTypeStr=Inherit: Same as first input
  Vitesse y7 : Integrator  InitialCondition=v_ini
  y7 : Outport  VectorParamsAs1DForOutWhenUnconnected=off
  vy7 : Outport  Port=2  VectorParamsAs1DForOutWhenUnconnected=off
  wires:
  Position y7/1 -> " "/1, y7/1
  Vitesse y7/1 -> Position y7/1, Product1/2, vy7/1
  Divide/1 -> Vitesse y7/1
  Somme Force/1 -> Divide/1
  Product1/1 -> Somme Force/3
  Fy7/1 -> Somme Force/2
  yp8/1 -> Somme y/3
  yp6/1 -> Somme y/2
  " "/1 -> Somme y/1
  b/1 -> Product1/1
  Somme y/1 -> Product2/1
  Product2/1 -> Somme Force/1
  k/1 -> Product2/2
  m/1 -> Divide/2

== system corde/corde /masse8 ==
  yp7 : Inport
  yp9 : Inport  Port=2
  Fy8 : Inport  Port=3
  b : Inport  Port=4
  k : Inport  Port=5
  m : Inport  Port=6
  " " : Gain  Gain=2  SaturateOnIntegerOverflow=on  OutDataTypeStr=Inherit: Same as input  ParamDataTypeStr=Inherit: Same as input
  Divide : Product  Inputs=*/
  Position y8 : Integrator  InitialCondition=pos_ini
  Product : Product
  Product1 : Product
  Somme Force : Sum  Inputs=++-  SaturateOnIntegerOverflow=on  InputSameDT=on  OutDataTypeStr=Inherit: Same as first input
  Somme y : Sum  Inputs=-++  SaturateOnIntegerOverflow=on  InputSameDT=on  OutDataTypeStr=Inherit: Same as first input
  Vitesse y8 : Integrator  InitialCondition=v_ini
  y8 : Outport  VectorParamsAs1DForOutWhenUnconnected=off
  vy8 : Outport  Port=2  VectorParamsAs1DForOutWhenUnconnected=off
  wires:
  Position y8/1 -> " "/1, y8/1
  Vitesse y8/1 -> Position y8/1, vy8/1, Product/1
  Divide/1 -> Vitesse y8/1
  Somme Force/1 -> Divide/1
  Product1/1 -> Somme Force/1
  Somme y/1 -> Product1/2
  Product/1 -> Somme Force/3
  Fy8/1 -> Somme Force/2
  yp9/1 -> Somme y/3
  yp7/1 -> Somme y/2
  " "/1 -> Somme y/1
  b/1 -> Product/2
  k/1 -> Product1/1
  m/1 -> Divide/2

== system corde/corde /masse9 ==
  yp8 : Inport
  yp10 : Inport  Port=2
  Fy9 : Inport  Port=3
  b : Inport  Port=4
  k : Inport  Port=5
  m : Inport  Port=6
  " " : Gain  Gain=2  SaturateOnIntegerOverflow=on  OutDataTypeStr=Inherit: Same as input  ParamDataTypeStr=Inherit: Same as input
  Divide : Product  Inputs=*/
  Position y9 : Integrator  InitialCondition=pos_ini
  Product : Product
  Product1 : Product
  Somme Force : Sum  Inputs=++-  SaturateOnIntegerOverflow=on  InputSameDT=on  OutDataTypeStr=Inherit: Same as first input
  Somme y : Sum  Inputs=-++  SaturateOnIntegerOverflow=on  InputSameDT=on  OutDataTypeStr=Inherit: Same as first input
  Vitesse y9 : Integrator  InitialCondition=v_ini
  y9 : Outport  VectorParamsAs1DForOutWhenUnconnected=off
  vy9 : Outport  Port=2  VectorParamsAs1DForOutWhenUnconnected=off
  wires:
  Position y9/1 -> " "/1, y9/1
  Vitesse y9/1 -> Position y9/1, Product/2, vy9/1
  Divide/1 -> Vitesse y9/1
  Somme Force/1 -> Divide/1
  Product1/1 -> Somme Force/1
  Somme y/1 -> Product1/2
  Product/1 -> Somme Force/3
  Fy9/1 -> Somme Force/2
  yp10/1 -> Somme y/3
  yp8/1 -> Somme y/2
  " "/1 -> Somme y/1
  b/1 -> Product/1
  k/1 -> Product1/1
  m/1 -> Divide/2
